simulink model "Mecanum_Mfunction_PID"  (R2022a)
settings: Solver=FixedStepAuto  StartTime=0.0  StopTime=20  FixedStep=0.001  RelTol=1e-3
values from neighbouring files (symbols this model uses):
  Cm = 0    [Mecanum_parameter_Mfunction_PID.m]
  Jm = 15.5*10^-7    (= 1.55e-06)    [Mecanum_parameter_Mfunction_PID.m]
  Kb = Kt    (= 0.0286)    [Mecanum_parameter_Mfunction_PID.m]
  Kf = 0    [Mecanum_parameter_Mfunction_PID.m]
  Kt = 28.6*10^-3    (= 0.0286)    [Mecanum_parameter_Mfunction_PID.m]
  La = 0.39*10^-3    (= 0.00039)    [Mecanum_parameter_Mfunction_PID.m]
  N = N_motor * N_wheel    (= 14)    [Mecanum_parameter_Mfunction_PID.m]
  Ra = 0.38    [Mecanum_parameter_Mfunction_PID.m]
libraries: simulink x1
(part 2 of 3)

== matlab function Mecanum_Mfunction_PID/Plant_Lagrange1/Lagrange_plant  ==
  settings: updateMethod=DISCRETE  sampleTime=0.001
  data: torque1 input; torque2 input; X_dotdot output; Y_dotdot output; Z_dotdot output; PHI_y_dotdot output; PHI_z_dotdot output; torque3 input; torque4 input; X_dot input; Y_dot input; Z_dot input; PHI_y_dot input; PHI_z_dot input; X input; Y input; Z input; PHI_y input; PHI_z input; X_dot output; Y_dot output; Z_dot output; PHI_y_dot output; PHI_z_dot output; X output; Y output; w1 input; w2 input; w3 input; w4 input; PHI_y output; PHI_z output
function [X_dotdot,Y_dotdot,Z_dotdot,PHI_y_dotdot,PHI_z_dotdot,X_dot,Y_dot,Z_dot,PHI_y_dot,PHI_z_dot,X,Y,PHI_y,PHI_z]  = fcn(torque1,torque2,torque3,torque4,X_dot,Y_dot,Z_dot,PHI_y_dot,PHI_z_dot,X,Y,Z,PHI_y,PHI_z,w1,w2,w3,w4)
%#codegen


%===== Parameter =====
%=== Body ===
m_b = 30; 
d = 0.6;
w = 0.4;
h = 1;
I_zb = 1/12*m_b*(d^2+w^2);
I_xb = 1/12*m_b*(h^2+d^2);
I_yb = 1/12*m_b*(w^2+h^2);

%=== Wheel ===
m_w = 0.4;
R = 0.05;
I_yw = m_w*R^2/2;
L_x_i = 0.2375;
L_y_i = 0.2394;
I_zw = m_w*(L_x_i^2+L_y_i^2);

%=== Friction ====
Friction = (m_b+4*m_w)/4*9.8*0.002;

if(w1>1)
    torque1 = torque1 - Friction;
else if(w1<-1)
    torque1 = torque1 + Friction;
    end
end

if(w2>1)
    torque2 = torque2 - Friction;
else if(w2<-1)
    torque2 = torque2 + Friction;
    end
end

if(w3>1)
    torque3 = torque3 - Friction;
else if(w3<-1)
    torque3 = torque3 + Friction;
    end
end

if(w4>1)
    torque4 = torque4 - Friction;
else if(w4<-1)
    torque4 = torque4 + Friction;
    end
end


dt = 0.001;
% 2D model

% Den_XY  = m_b + 4*m_w + 4*(I_yw/(R^2));
% Den_PHI = I_zb + 4*I_zw + 4*m_w*(Lx^2+Ly^2) + 4*I_yw/(R^2)*(Lx+Ly)^2 ;
% 
% Buff_X   = (cos(PHI)+sin(PHI))/R*(torque1+torque4) + (cos(PHI)-sin(PHI))/R*(torque2+torque3) - 4*I_yw/(R^2)*Y_dot*PHI_dot;
% Buff_Y   = (sin(PHI)-cos(PHI))/R*(torque1+torque4) + (sin(PHI)+cos(PHI))/R*(torque2+torque3) + 4*I_yw/(R^2)*X_dot*PHI_dot;
% Buff_PHI = (Lx+Ly)/R*(-torque1+torque2-torque3+torque4);

% X_dotdot   = Buff_X/Den_XY;
% Y_dotdot   = Buff_Y/Den_XY;
% PHI_dotdot = Buff_PHI/Den_PHI;
%%%%
X_dotdot = (32*G*I_yw^3*R^2*sin(2*PHI_y) - 32*G*I_yw^3*L_z_i^2*sin(2*PHI_y) + 8*G*I_yw^2*R^4*m_b*sin(2*PHI_y) + 32*G*I_yw^2*R^4*m_w*sin(2*PHI_y) + 16*I_yw^2*L_z_i^2*R^3*torque1*cos(PHI_z) + 16*I_yw^2*L_z_i^2*R^3*torque2*cos(PHI_z) + 16*I_yw^2*L_z_i^2*R^3*torque3*cos(PHI_z) + 16*I_yw^2*L_z_i^2*R^3*torque4*cos(PHI_z) + 64*I_yw^3*L_z_i^2*cos(PHI_y)*Y_dot*PHI_z_dot - 64*I_yw^3*R^2*cos(PHI_y)*Y_dot*PHI_z_dot + 32*G*I_yw^3*L_z_i^2*R^2*sin(2*PHI_y) - 64*I_yw^3*L_z_i^2*cos(PHI_y)^2*Z_dot*PHI_y_dot + 16*I_yw^2*R^3*torque1*cos(PHI_y)*cos(PHI_z) + 16*I_yw^2*R^3*torque2*cos(PHI_y)*cos(PHI_z) + 16*I_yw^2*R^3*torque3*cos(PHI_y)*cos(PHI_z) + 16*I_yw^2*R^3*torque4*cos(PHI_y)*cos(PHI_z) + 64*I_yw^3*R^2*cos(PHI_y)^2*Z_dot*PHI_y_dot - 32*I_yw^3*L_z_i^2*sin(2*PHI_y)*X_dot*PHI_y_dot + 32*I_yw^3*R^2*sin(2*PHI_y)*X_dot*PHI_y_dot + 16*I_yw^2*R^3*torque1*cos(PHI_y)*sin(PHI_z) - 16*I_yw^2*R^3*torque2*cos(PHI_y)*sin(PHI_z) - 16*I_yw^2*R^3*torque3*cos(PHI_y)*sin(PHI_z) + 16*I_yw^2*R^3*torque4*cos(PHI_y)*sin(PHI_z) + 8*G*I_yb*I_yw^2*R^2*sin(2*PHI_y) + 2*G*I_yb*I_yw*R^4*m_b*sin(2*PHI_y) + 8*G*I_yb*I_yw*R^4*m_w*sin(2*PHI_y) - 16*I_yw^2*L_z_i^2*R*torque1*cos(PHI_y)*sin(PHI_z) + 16*I_yw^2*L_z_i^2*R*torque2*cos(PHI_y)*sin(PHI_z) + 16*I_yw^2*L_z_i^2*R*torque3*cos(PHI_y)*sin(PHI_z) - 16*I_yw^2*L_z_i^2*R*torque4*cos(PHI_y)*sin(PHI_z) + 16*I_yw^2*L_z_i^2*R^3*torque1*cos(PHI_y)^2*cos(PHI_z)^3 + 16*I_yw^2*L_z_i^2*R^3*torque2*cos(PHI_y)^2*cos(PHI_z)^3 + 16*I_yw^2*L_z_i^2*R^3*torque3*cos(PHI_y)^2*cos(PHI_z)^3 + 16*I_yw^2*L_z_i^2*R^3*torque4*cos(PHI_y)^2*cos(PHI_z)^3 + 16*I_yw^2*R^4*m_b*cos(PHI_y)^2*Z_dot*PHI_y_dot + 64*I_yw^2*R^4*m_w*cos(PHI_y)^2*Z_dot*PHI_y_dot + 8*I_yw^2*R^4*m_b*sin(2*PHI_y)*X_dot*PHI_y_dot + 32*I_yw^2*R^4*m_w*sin(2*PHI_y)*X_dot*PHI_y_dot + 4*I_yw*L_z_i^2*R^5*m_b*torque1*cos(PHI_z) + 4*I_yw*L_z_i^2*R^5*m_b*torque2*cos(PHI_z) + 4*I_yw*L_z_i^2*R^5*m_b*torque3*cos(PHI_z) + 4*I_yw*L_z_i^2*R^5*m_b*torque4*cos(PHI_z) + 16*I_yw*L_z_i^2*R^5*m_w*torque1*cos(PHI_z) + 16*I_yw*L_z_i^2*R^5*m_w*torque2*cos(PHI_z) + 16*I_yw*L_z_i^2*R^5*m_w*torque3*cos(PHI_z) + 16*I_yw*L_z_i^2*R^5*m_w*torque4*cos(PHI_z) + 16*I_yw^2*L_z_i^2*R^3*torque1*cos(PHI_y)*cos(PHI_z) + 16*I_yw^2*L_z_i^2*R^3*torque2*cos(PHI_y)*cos(PHI_z) + 16*I_yw^2*L_z_i^2*R^3*torque3*cos(PHI_y)*cos(PHI_z) + 16*I_yw^2*L_z_i^2*R^3*torque4*cos(PHI_y)*cos(PHI_z) + 64*I_yw^3*L_z_i^2*R^2*cos(PHI_y)^2*Z_dot*PHI_y_dot - 64*I_yw^3*L_z_i^2*R^2*cos(PHI_z)^2*Y_dot*PHI_z_dot + 32*I_yw^3*L_z_i^2*R^2*sin(2*PHI_y)*X_dot*PHI_y_dot + 16*I_yw^2*L_z_i^2*R^3*torque1*cos(PHI_y)*sin(PHI_z) - 16*I_yw^2*L_z_i^2*R^3*torque2*cos(PHI_y)*sin(PHI_z) - 16*I_yw^2*L_z_i^2*R^3*torque3*cos(PHI_y)*sin(PHI_z) + 16*I_yw^2*L_z_i^2*R^3*torque4*cos(PHI_y)*sin(PHI_z) + 16*L_x_i^2*R^5*m_w^2*torque1*cos(PHI_y)*cos(PHI_z) + 16*L_x_i^2*R^5*m_w^2*torque2*cos(PHI_y)*cos(PHI_z) + 16*L_x_i^2*R^5*m_w^2*torque3*cos(PHI_y)*cos(PHI_z) + 16*L_x_i^2*R^5*m_w^2*torque4*cos(PHI_y)*cos(PHI_z) + 16*L_y_i^2*R^5*m_w^2*torque1*cos(PHI_y)*cos(PHI_z) + 16*L_y_i^2*R^5*m_w^2*torque2*cos(PHI_y)*cos(PHI_z) + 16*L_y_i^2*R^5*m_w^2*torque3*cos(PHI_y)*cos(PHI_z) + 16*L_y_i^2*R^5*m_w^2*torque4*cos(PHI_y)*cos(PHI_z) + 16*L_z_i^2*R^5*m_w^2*torque1*cos(PHI_y)*cos(PHI_z) + 16*L_z_i^2*R^5*m_w^2*torque2*cos(PHI_y)*cos(PHI_z) + 16*L_z_i^2*R^5*m_w^2*torque3*cos(PHI_y)*cos(PHI_z) + 16*L_z_i^2*R^5*m_w^2*torque4*cos(PHI_y)*cos(PHI_z) + 16*L_x_i^2*R^5*m_w^2*torque1*cos(PHI_y)*sin(PHI_z) - 16*L_x_i^2*R^5*m_w^2*torque2*cos(PHI_y)*sin(PHI_z) - 16*L_x_i^2*R^5*m_w^2*torque3*cos(PHI_y)*sin(PHI_z) + 16*L_x_i^2*R^5*m_w^2*torque4*cos(PHI_y)*sin(PHI_z) + 16*L_y_i^2*R^5*m_w^2*torque1*cos(PHI_y)*sin(PHI_z) - 16*L_y_i^2*R^5*m_w^2*torque2*cos(PHI_y)*sin(PHI_z) - 16*L_y_i^2*R^5*m_w^2*torque3*cos(PHI_y)*sin(PHI_z) + 16*L_y_i^2*R^5*m_w^2*torque4*cos(PHI_y)*sin(PHI_z) + 16*L_z_i^2*R^5*m_w^2*torque1*cos(PHI_y)*sin(PHI_z) - 16*L_z_i^2*R^5*m_w^2*torque2*cos(PHI_y)*sin(PHI_z) - 16*L_z_i^2*R^5*m_w^2*torque3*cos(PHI_y)*sin(PHI_z) + 16*L_z_i^2*R^5*m_w^2*torque4*cos(PHI_y)*sin(PHI_z) + 4*I_yb*I_yw*R^3*torque1*cos(PHI_y)*cos(PHI_z) + 4*I_yb*I_yw*R^3*torque2*cos(PHI_y)*cos(PHI_z) + 4*I_yb*I_yw*R^3*torque3*cos(PHI_y)*cos(PHI_z) + 4*I_yb*I_yw*R^3*torque4*cos(PHI_y)*cos(PHI_z) + 64*G*I_yw^3*L_z_i^2*R^2*cos(PHI_z)^2*sin(PHI_y) - 16*I_yb*I_yw^2*R^2*cos(PHI_y)*Y_dot*PHI_z_dot + 4*I_yb*I_yw*R^3*torque1*cos(PHI_y)*sin(PHI_z) - 4*I_yb*I_yw*R^3*torque2*cos(PHI_y)*sin(PHI_z) - 4*I_yb*I_yw*R^3*torque3*cos(PHI_y)*sin(PHI_z) + 4*I_yb*I_yw*R^3*torque4*cos(PHI_y)*sin(PHI_z) - 16*I_yw^2*L_z_i^2*R^3*torque1*cos(PHI_y)^2*cos(PHI_z) - 16*I_yw^2*L_z_i^2*R^3*torque1*cos(PHI_y)*cos(PHI_z)^3 - 16*I_yw^2*L_z_i^2*R^3*torque2*cos(PHI_y)^2*cos(PHI_z) - 16*I_yw^2*L_z_i^2*R^3*torque2*cos(PHI_y)*cos(PHI_z)^3 - 16*I_yw^2*L_z_i^2*R^3*torque3*cos(PHI_y)^2*cos(PHI_z) - 16*I_yw^2*L_z_i^2*R^3*torque3*cos(PHI_y)*cos(PHI_z)^3 - 16*I_yw^2*L_z_i^2*R^3*torque4*cos(PHI_y)^2*cos(PHI_z) - 16*I_yw^2*L_z_i^2*R^3*torque4*cos(PHI_y)*cos(PHI_z)^3 + I_yb*R^5*m_b*torque1*cos(PHI_y)*cos(PHI_z) + I_yb*R^5*m_b*torque2*cos(PHI_y)*cos(PHI_z) + I_yb*R^5*m_b*torque3*cos(PHI_y)*cos(PHI_z) + I_yb*R^5*m_b*torque4*cos(PHI_y)*cos(PHI_z) + 4*I_yw*R^5*m_b*torque1*cos(PHI_y)*cos(PHI_z) + 4*I_yw*R^5*m_b*torque2*cos(PHI_y)*cos(PHI_z) + 4*I_yw*R^5*m_b*torque3*cos(PHI_y)*cos(PHI_z) + 4*I_yw*R^5*m_b*torque4*cos(PHI_y)*cos(PHI_z) + 4*I_yb*R^5*m_w*torque1*cos(PHI_y)*cos(PHI_z) + 4*I_yb*R^5*m_w*torque2*cos(PHI_y)*cos(PHI_z) + 4*I_yb*R^5*m_w*torque3*cos(PHI_y)*cos(PHI_z) + 4*I_yb*R^5*m_w*torque4*cos(PHI_y)*cos(PHI_z) + 16*I_yw*R^5*m_w*torque1*cos(PHI_y)*cos(PHI_z) + 16*I_yw*R^5*m_w*torque2*cos(PHI_y)*cos(PHI_z) + 16*I_yw*R^5*m_w*torque3*cos(PHI_y)*cos(PHI_z) + 16*I_yw*R^5*m_w*torque4*cos(PHI_y)*cos(PHI_z) - 16*I_yw^2*R^4*m_b*cos(PHI_y)*Y_dot*PHI_z_dot - 64*I_yw^2*R^4*m_w*cos(PHI_y)*Y_dot*PHI_z_dot - 8*G*I_yw^2*L_z_i^2*R^2*m_b*sin(2*PHI_y) + 32*G*I_yw^2*L_x_i^2*R^2*m_w*sin(2*PHI_y) + 32*G*I_yw*L_x_i^2*R^4*m_w^2*sin(2*PHI_y) + 32*G*I_yw^2*L_y_i^2*R^2*m_w*sin(2*PHI_y) + 32*G*I_yw*L_y_i^2*R^4*m_w^2*sin(2*PHI_y) + 32*G*I_yw*L_z_i^2*R^4*m_w^2*sin(2*PHI_y) + I_yb*R^5*m_b*torque1*cos(PHI_y)*sin(PHI_z) - I_yb*R^5*m_b*torque2*cos(PHI_y)*sin(PHI_z) - I_yb*R^5*m_b*torque3*cos(PHI_y)*sin(PHI_z) + I_yb*R^5*m_b*torque4*cos(PHI_y)*sin(PHI_z) + 4*I_yw*R^5*m_b*torque1*cos(PHI_y)*sin(PHI_z) - 4*I_yw*R^5*m_b*torque2*cos(PHI_y)*sin(PHI_z) - 4*I_yw*R^5*m_b*torque3*cos(PHI_y)*sin(PHI_z) + 4*I_yw*R^5*m_b*torque4*cos(PHI_y)*sin(PHI_z) + 4*I_yb*R^5*m_w*torque1*cos(PHI_y)*sin(PHI_z) - 4*I_yb*R^5*m_w*torque2*cos(PHI_y)*sin(PHI_z) - 4*I_yb*R^5*m_w*torque3*cos(PHI_y)*sin(PHI_z) + 4*I_yb*R^5*m_w*torque4*cos(PHI_y)*sin(PHI_z) + 16*I_yw*R^5*m_w*torque1*cos(PHI_y)*sin(PHI_z) - 16*I_yw*R^5*m_w*torque2*cos(PHI_y)*sin(PHI_z) - 16*I_yw*R^5*m_w*torque3*cos(PHI_y)*sin(PHI_z) + 16*I_yw*R^5*m_w*torque4*cos(PHI_y)*sin(PHI_z) + 16*I_yb*I_yw^2*R^2*cos(PHI_y)^2*Z_dot*PHI_y_dot - 16*I_yw^2*L_z_i^2*R*torque1*cos(PHI_y)*cos(PHI_z) - 16*I_yw^2*L_z_i^2*R*torque2*cos(PHI_y)*cos(PHI_z) - 16*I_yw^2*L_z_i^2*R*torque3*cos(PHI_y)*cos(PHI_z) - 16*I_yw^2*L_z_i^2*R*torque4*cos(PHI_y)*cos(PHI_z) - 64*I_yw^3*L_z_i^2*R^2*cos(PHI_y)*Y_dot*PHI_z_dot + 8*I_yb*I_yw^2*R^2*sin(2*PHI_y)*X_dot*PHI_y_dot - 16*I_yw^2*L_z_i^2*R^3*torque1*cos(PHI_y)*cos(PHI_z)^2*sin(PHI_z) + 16*I_yw^2*L_z_i^2*R^3*torque2*cos(PHI_y)*cos(PHI_z)^2*sin(PHI_z) + 16*I_yw^2*L_z_i^2*R^3*torque3*cos(PHI_y)*cos(PHI_z)^2*sin(PHI_z) - 16*I_yw^2*L_z_i^2*R^3*torque4*cos(PHI_y)*cos(PHI_z)^2*sin(PHI_z) + 16*G*I_yw^2*L_z_i^2*R^4*m_b*cos(PHI_z)^2*sin(PHI_y) + 64*G*I_yw^2*L_z_i^2*R^4*m_w*cos(PHI_z)^2*sin(PHI_y) + 2*I_yb*I_yw*R^4*m_b*sin(2*PHI_y)*X_dot*PHI_y_dot + 8*I_yb*I_yw*R^4*m_w*sin(2*PHI_y)*X_dot*PHI_y_dot + 16*I_yw^2*L_z_i^2*R^3*torque1*cos(PHI_y)^2*cos(PHI_z)^2*sin(PHI_z) - 16*I_yw^2*L_z_i^2*R^3*torque2*cos(PHI_y)^2*cos(PHI_z)^2*sin(PHI_z) - 16*I_yw^2*L_z_i^2*R^3*torque3*cos(PHI_y)^2*cos(PHI_z)^2*sin(PHI_z) + 16*I_yw^2*L_z_i^2*R^3*torque4*cos(PHI_y)^2*cos(PHI_z)^2*sin(PHI_z) - 4*I_yw*L_z_i^2*R^3*m_b*torque1*cos(PHI_y)*cos(PHI_z) - 4*I_yw*L_z_i^2*R^3*m_b*torque2*cos(PHI_y)*cos(PHI_z) - 4*I_yw*L_z_i^2*R^3*m_b*torque3*cos(PHI_y)*cos(PHI_z) - 4*I_yw*L_z_i^2*R^3*m_b*torque4*cos(PHI_y)*cos(PHI_z) + 16*I_yw*L_x_i^2*R^3*m_w*torque1*cos(PHI_y)*cos(PHI_z) + 16*I_yw*L_x_i^2*R^3*m_w*torque2*cos(PHI_y)*cos(PHI_z) + 16*I_yw*L_x_i^2*R^3*m_w*torque3*cos(PHI_y)*cos(PHI_z) + 16*I_yw*L_x_i^2*R^3*m_w*torque4*cos(PHI_y)*cos(PHI_z) + 16*I_yw*L_y_i^2*R^3*m_w*torque1*cos(PHI_y)*cos(PHI_z) + 16*I_yw*L_y_i^2*R^3*m_w*torque2*cos(PHI_y)*cos(PHI_z) + 16*I_yw*L_y_i^2*R^3*m_w*torque3*cos(PHI_y)*cos(PHI_z) + 16*I_yw*L_y_i^2*R^3*m_w*torque4*cos(PHI_y)*cos(PHI_z) + 16*I_yw^2*L_z_i^2*R^2*m_b*cos(PHI_y)*Y_dot*PHI_z_dot - 64*I_yw^2*L_x_i^2*R^2*m_w*cos(PHI_y)*Y_dot*PHI_z_dot - 64*I_yw*L_x_i^2*R^4*m_w^2*cos(PHI_y)*Y_dot*PHI_z_dot - 64*I_yw^2*L_y_i^2*R^2*m_w*cos(PHI_y)*Y_dot*PHI_z_dot - 64*I_yw*L_y_i^2*R^4*m_w^2*cos(PHI_y)*Y_dot*PHI_z_dot - 64*I_yw*L_z_i^2*R^4*m_w^2*cos(PHI_y)*Y_dot*PHI_z_dot - 4*I_yw*L_z_i^2*R^3*m_b*torque1*cos(PHI_y)*sin(PHI_z) + 4*I_yw*L_z_i^2*R^3*m_b*torque2*cos(PHI_y)*sin(PHI_z) + 4*I_yw*L_z_i^2*R^3*m_b*torque3*cos(PHI_y)*sin(PHI_z) - 4*I_yw*L_z_i^2*R^3*m_b*torque4*cos(PHI_y)*sin(PHI_z) + 16*I_yw*L_x_i^2*R^3*m_w*torque1*cos(PHI_y)*sin(PHI_z) - 16*I_yw*L_x_i^2*R^3*m_w*torque2*cos(PHI_y)*sin(PHI_z) - 16*I_yw*L_x_i^2*R^3*m_w*torque3*cos(PHI_y)*sin(PHI_z) + 16*I_yw*L_x_i^2*R^3*m_w*torque4*cos(PHI_y)*sin(PHI_z) + 16*I_yw*L_y_i^2*R^3*m_w*torque1*cos(PHI_y)*sin(PHI_z) - 16*I_yw*L_y_i^2*R^3*m_w*torque2*cos(PHI_y)*sin(PHI_z) - 16*I_yw*L_y_i^2*R^3*m_w*torque3*cos(PHI_y)*sin(PHI_z) + 16*I_yw*L_y_i^2*R^3*m_w*torque4*cos(PHI_y)*sin(PHI_z) + 4*L_x_i^2*R^5*m_b*m_w*torque1*cos(PHI_y)*cos(PHI_z) + 4*L_x_i^2*R^5*m_b*m_w*torque2*cos(PHI_y)*cos(PHI_z) + 4*L_x_i^2*R^5*m_b*m_w*torque3*cos(PHI_y)*cos(PHI_z) + 4*L_x_i^2*R^5*m_b*m_w*torque4*cos(PHI_y)*cos(PHI_z) + 4*L_y_i^2*R^5*m_b*m_w*torque1*cos(PHI_y)*cos(PHI_z) + 4*L_y_i^2*R^5*m_b*m_w*torque2*cos(PHI_y)*cos(PHI_z) + 4*L_y_i^2*R^5*m_b*m_w*torque3*cos(PHI_y)*cos(PHI_z) + 4*L_y_i^2*R^5*m_b*m_w*torque4*cos(PHI_y)*cos(PHI_z) + 4*L_z_i^2*R^5*m_b*m_w*torque1*cos(PHI_y)*cos(PHI_z) + 4*L_z_i^2*R^5*m_b*m_w*torque2*cos(PHI_y)*cos(PHI_z) + 4*L_z_i^2*R^5*m_b*m_w*torque3*cos(PHI_y)*cos(PHI_z) + 4*L_z_i^2*R^5*m_b*m_w*torque4*cos(PHI_y)*cos(PHI_z) + 64*I_yw^3*L_z_i^2*R^2*cos(PHI_y)*cos(PHI_z)^2*Z_dot*PHI_y_dot + 4*L_x_i^2*R^5*m_b*m_w*torque1*cos(PHI_y)*sin(PHI_z) - 4*L_x_i^2*R^5*m_b*m_w*torque2*cos(PHI_y)*sin(PHI_z) - 4*L_x_i^2*R^5*m_b*m_w*torque3*cos(PHI_y)*sin(PHI_z) + 4*L_x_i^2*R^5*m_b*m_w*torque4*cos(PHI_y)*sin(PHI_z) + 4*L_y_i^2*R^5*m_b*m_w*torque1*cos(PHI_y)*sin(PHI_z) - 4*L_y_i^2*R^5*m_b*m_w*torque2*cos(PHI_y)*sin(PHI_z) - 4*L_y_i^2*R^5*m_b*m_w*torque3*cos(PHI_y)*sin(PHI_z) + 4*L_y_i^2*R^5*m_b*m_w*torque4*cos(PHI_y)*sin(PHI_z) + 4*L_z_i^2*R^5*m_b*m_w*torque1*cos(PHI_y)*sin(PHI_z) - 4*L_z_i^2*R^5*m_b*m_w*torque2*cos(PHI_y)*sin(PHI_z) - 4*L_z_i^2*R^5*m_b*m_w*torque3*cos(PHI_y)*sin(PHI_z) + 4*L_z_i^2*R^5*m_b*m_w*torque4*cos(PHI_y)*sin(PHI_z) + 64*I_yw^3*L_z_i^2*R^2*cos(PHI_y)*cos(PHI_z)^2*Y_dot*PHI_z_dot + 16*I_yw^2*L_z_i^2*R^3*torque1*cos(PHI_y)*cos(PHI_z)*sin(PHI_y) + 16*I_yw^2*L_z_i^2*R^3*torque2*cos(PHI_y)*cos(PHI_z)*sin(PHI_y) + 16*I_yw^2*L_z_i^2*R^3*torque3*cos(PHI_y)*cos(PHI_z)*sin(PHI_y) + 16*I_yw^2*L_z_i^2*R^3*torque4*cos(PHI_y)*cos(PHI_z)*sin(PHI_y) + 64*I_yw^3*L_z_i^2*R^2*cos(PHI_z)^2*sin(PHI_y)*X_dot*PHI_y_dot - 4*I_yb*I_yw*R^4*m_b*cos(PHI_y)*Y_dot*PHI_z_dot - 16*I_yb*I_yw*R^4*m_w*cos(PHI_y)*Y_dot*PHI_z_dot - 16*I_yw^2*L_z_i^2*R^2*m_b*cos(PHI_y)^2*Z_dot*PHI_y_dot + 64*I_yw^2*L_x_i^2*R^2*m_w*cos(PHI_y)^2*Z_dot*PHI_y_dot + 64*I_yw*L_x_i^2*R^4*m_w^2*cos(PHI_y)^2*Z_dot*PHI_y_dot + 64*I_yw^2*L_y_i^2*R^2*m_w*cos(PHI_y)^2*Z_dot*PHI_y_dot + 64*I_yw*L_y_i^2*R^4*m_w^2*cos(PHI_y)^2*Z_dot*PHI_y_dot + 64*I_yw*L_z_i^2*R^4*m_w^2*cos(PHI_y)^2*Z_dot*PHI_y_dot - 16*I_yw^2*L_z_i^2*R^4*m_b*cos(PHI_z)^2*Y_dot*PHI_z_dot - 64*I_yw^2*L_z_i^2*R^4*m_w*cos(PHI_z)^2*Y_dot*PHI_z_dot - 64*G*I_yw^3*L_z_i^2*R^2*cos(PHI_y)*cos(PHI_z)^2*sin(PHI_y) - 8*I_yw^2*L_z_i^2*R^2*m_b*sin(2*PHI_y)*X_dot*PHI_y_dot + 32*I_yw^2*L_x_i^2*R^2*m_w*sin(2*PHI_y)*X_dot*PHI_y_dot + 32*I_yw*L_x_i^2*R^4*m_w^2*sin(2*PHI_y)*X_dot*PHI_y_dot + 32*I_yw^2*L_y_i^2*R^2*m_w*sin(2*PHI_y)*X_dot*PHI_y_dot + 32*I_yw*L_y_i^2*R^4*m_w^2*sin(2*PHI_y)*X_dot*PHI_y_dot + 32*I_yw*L_z_i^2*R^4*m_w^2*sin(2*PHI_y)*X_dot*PHI_y_dot + 8*G*I_yw*L_x_i^2*R^4*m_b*m_w*sin(2*PHI_y) + 8*G*I_yw*L_y_i^2*R^4*m_b*m_w*sin(2*PHI_y) + 8*G*I_yw*L_z_i^2*R^4*m_b*m_w*sin(2*PHI_y) - 64*I_yw^3*L_z_i^2*R^2*cos(PHI_y)^2*cos(PHI_z)^2*Z_dot*PHI_y_dot - 16*I_yw^2*L_z_i^2*R^3*torque1*cos(PHI_y)*cos(PHI_z)^3*sin(PHI_y) - 16*I_yw^2*L_z_i^2*R^3*torque2*cos(PHI_y)*cos(PHI_z)^3*sin(PHI_y) - 16*I_yw^2*L_z_i^2*R^3*torque3*cos(PHI_y)*cos(PHI_z)^3*sin(PHI_y) - 16*I_yw^2*L_z_i^2*R^3*torque4*cos(PHI_y)*cos(PHI_z)^3*sin(PHI_y) + 4*I_yb*I_yw*R^4*m_b*cos(PHI_y)^2*Z_dot*PHI_y_dot + 16*I_yb*I_yw*R^4*m_w*cos(PHI_y)^2*Z_dot*PHI_y_dot + 16*I_yw^2*L_z_i^2*R^4*m_b*cos(PHI_y)*cos(PHI_z)^2*Z_dot*PHI_y_dot + 64*I_yw^2*L_z_i^2*R^4*m_w*cos(PHI_y)*cos(PHI_z)^2*Z_dot*PHI_y_dot + 16*I_yw^2*L_z_i^2*R^4*m_b*cos(PHI_z)^2*sin(PHI_y)*X_dot*PHI_y_dot + 64*I_yw^2*L_z_i^2*R^4*m_w*cos(PHI_z)^2*sin(PHI_y)*X_dot*PHI_y_dot - 16*I_yw^2*L_z_i^2*R^3*torque1*cos(PHI_y)*cos(PHI_z)^2*sin(PHI_y)*sin(PHI_z) + 16*I_yw^2*L_z_i^2*R^3*torque2*cos(PHI_y)*cos(PHI_z)^2*sin(PHI_y)*sin(PHI_z) + 16*I_yw^2*L_z_i^2*R^3*torque3*cos(PHI_y)*cos(PHI_z)^2*sin(PHI_y)*sin(PHI_z) - 16*I_yw^2*L_z_i^2*R^3*torque4*cos(PHI_y)*cos(PHI_z)^2*sin(PHI_y)*sin(PHI_z) - 16*I_yw*L_x_i^2*R^4*m_b*m_w*cos(PHI_y)*Y_dot*PHI_z_dot - 16*I_yw*L_y_i^2*R^4*m_b*m_w*cos(PHI_y)*Y_dot*PHI_z_dot - 16*I_yw*L_z_i^2*R^4*m_b*m_w*cos(PHI_y)*Y_dot*PHI_z_dot + 64*I_yw^3*L_z_i^2*R^2*cos(PHI_y)*cos(PHI_z)*sin(PHI_z)*X_dot*PHI_z_dot - 64*I_yw^3*L_z_i^2*R^2*cos(PHI_y)*cos(PHI_z)*sin(PHI_z)*Z_dot*PHI_z_dot - 64*I_yw^3*L_z_i^2*R^2*cos(PHI_z)*sin(PHI_y)*sin(PHI_z)*Z_dot*PHI_z_dot + 16*I_yw*L_x_i^2*R^4*m_b*m_w*cos(PHI_y)^2*Z_dot*PHI_y_dot + 16*I_yw*L_y_i^2*R^4*m_b*m_w*cos(PHI_y)^2*Z_dot*PHI_y_dot + 16*I_yw*L_z_i^2*R^4*m_b*m_w*cos(PHI_y)^2*Z_dot*PHI_y_dot - 64*I_yw^3*L_z_i^2*R^2*cos(PHI_y)*cos(PHI_z)^2*sin(PHI_y)*X_dot*PHI_y_dot + 8*I_yw*L_x_i^2*R^4*m_b*m_w*sin(2*PHI_y)*X_dot*PHI_y_dot + 8*I_yw*L_y_i^2*R^4*m_b*m_w*sin(2*PHI_y)*X_dot*PHI_y_dot + 8*I_yw*L_z_i^2*R^4*m_b*m_w*sin(2*PHI_y)*X_dot*PHI_y_dot - 64*I_yw^3*L_z_i^2*R^2*cos(PHI_y)^3*cos(PHI_z)*sin(PHI_z)*X_dot*PHI_z_dot + 64*I_yw^3*L_z_i^2*R^2*cos(PHI_y)^3*cos(PHI_z)*sin(PHI_z)*Z_dot*PHI_z_dot - 16*I_yw^2*L_z_i^2*R^4*m_b*cos(PHI_z)*sin(PHI_y)*sin(PHI_z)*Z_dot*PHI_z_dot - 64*I_yw^2*L_z_i^2*R^4*m_w*cos(PHI_z)*sin(PHI_y)*sin(PHI_z)*Z_dot*PHI_z_dot + 64*I_yw^3*L_z_i^2*R^2*cos(PHI_y)^2*cos(PHI_z)*sin(PHI_y)*sin(PHI_z)*X_dot*PHI_z_dot + 64*I_yw^3*L_z_i^2*R^2*cos(PHI_y)^2*cos(PHI_z)*sin(PHI_y)*sin(PHI_z)*Z_dot*PHI_z_dot + 16*I_yw^2*L_z_i^2*R^4*m_b*cos(PHI_y)*cos(PHI_z)*sin(PHI_z)*X_dot*PHI_z_dot + 64*I_yw^2*L_z_i^2*R^4*m_w*cos(PHI_y)*cos(PHI_z)*sin(PHI_z)*X_dot*PHI_z_dot)/((4*I_yw + R^2*m_b + 4*R^2*m_w)*(16*I_yw^2*R^2 - 16*I_yw^2*L_z_i^2 + 16*I_yw^2*L_z_i^2*R^2 + 16*L_x_i^2*R^4*m_w^2 + 16*L_y_i^2*R^4*m_w^2 + 16*L_z_i^2*R^4*m_w^2 + 4*I_yb*I_yw*R^2 + I_yb*R^4*m_b + 4*I_yw*R^4*m_b + 4*I_yb*R^4*m_w + 16*I_yw*R^4*m_w - 16*I_yw^2*L_z_i^2*R^2*cos(PHI_z)^2 - 4*I_yw*L_z_i^2*R^2*m_b + 16*I_yw*L_x_i^2*R^2*m_w + 16*I_yw*L_y_i^2*R^2*m_w + 4*L_x_i^2*R^4*m_b*m_w + 4*L_y_i^2*R^4*m_b*m_w + 4*L_z_i^2*R^4*m_b*m_w + 16*I_yw^2*L_z_i^2*R^2*cos(PHI_y)*cos(PHI_z)^2 - 16*I_yw^2*L_z_i^2*R^2*cos(PHI_z)^2*sin(PHI_y)));
Y_dotdot = (16*I_yw^2*R^3*torque2*cos(PHI_z) - 16*I_yw^2*R^3*torque1*cos(PHI_z) + 16*I_yw^2*R^3*torque3*cos(PHI_z) - 16*I_yw^2*R^3*torque4*cos(PHI_z) + 16*I_yw^2*R^3*torque1*sin(PHI_z) + 16*I_yw^2*R^3*torque2*sin(PHI_z) + 16*I_yw^2*R^3*torque3*sin(PHI_z) + 16*I_yw^2*R^3*torque4*sin(PHI_z) - 16*I_yw^2*L_z_i^2*R^3*torque1*cos(PHI_z) + 16*I_yw^2*L_z_i^2*R^3*torque2*cos(PHI_z) + 16*I_yw^2*L_z_i^2*R^3*torque3*cos(PHI_z) - 16*I_yw^2*L_z_i^2*R^3*torque4*cos(PHI_z) - 16*L_x_i^2*R^5*m_w^2*torque1*cos(PHI_z) + 16*L_x_i^2*R^5*m_w^2*torque2*cos(PHI_z) + 16*L_x_i^2*R^5*m_w^2*torque3*cos(PHI_z) - 16*L_x_i^2*R^5*m_w^2*torque4*cos(PHI_z) - 16*L_y_i^2*R^5*m_w^2*torque1*cos(PHI_z) + 16*L_y_i^2*R^5*m_w^2*torque2*cos(PHI_z) + 16*L_y_i^2*R^5*m_w^2*torque3*cos(PHI_z) - 16*L_y_i^2*R^5*m_w^2*torque4*cos(PHI_z) - 16*L_z_i^2*R^5*m_w^2*torque1*cos(PHI_z) + 16*L_z_i^2*R^5*m_w^2*torque2*cos(PHI_z) + 16*L_z_i^2*R^5*m_w^2*torque3*cos(PHI_z) - 16*L_z_i^2*R^5*m_w^2*torque4*cos(PHI_z) - 64*I_yw^3*L_z_i^2*cos(PHI_y)*X_dot*PHI_z_dot + 64*I_yw^3*R^2*cos(PHI_y)*X_dot*PHI_z_dot + 16*L_x_i^2*R^5*m_w^2*torque1*sin(PHI_z) + 16*L_x_i^2*R^5*m_w^2*torque2*sin(PHI_z) + 16*L_x_i^2*R^5*m_w^2*torque3*sin(PHI_z) + 16*L_x_i^2*R^5*m_w^2*torque4*sin(PHI_z) + 16*L_y_i^2*R^5*m_w^2*torque1*sin(PHI_z) + 16*L_y_i^2*R^5*m_w^2*torque2*sin(PHI_z) + 16*L_y_i^2*R^5*m_w^2*torque3*sin(PHI_z) + 16*L_y_i^2*R^5*m_w^2*torque4*sin(PHI_z) + 16*L_z_i^2*R^5*m_w^2*torque1*sin(PHI_z) + 16*L_z_i^2*R^5*m_w^2*torque2*sin(PHI_z) + 16*L_z_i^2*R^5*m_w^2*torque3*sin(PHI_z) + 16*L_z_i^2*R^5*m_w^2*torque4*sin(PHI_z) - 4*I_yb*I_yw*R^3*torque1*cos(PHI_z) + 4*I_yb*I_yw*R^3*torque2*cos(PHI_z) + 4*I_yb*I_yw*R^3*torque3*cos(PHI_z) - 4*I_yb*I_yw*R^3*torque4*cos(PHI_z) + 64*I_yw^3*L_z_i^2*sin(PHI_y)*Z_dot*PHI_z_dot - 64*I_yw^3*R^2*sin(PHI_y)*Z_dot*PHI_z_dot + 4*I_yb*I_yw*R^3*torque1*sin(PHI_z) + 4*I_yb*I_yw*R^3*torque2*sin(PHI_z) + 4*I_yb*I_yw*R^3*torque3*sin(PHI_z) + 4*I_yb*I_yw*R^3*torque4*sin(PHI_z) + 16*I_yw^2*L_z_i^2*R^3*torque1*cos(PHI_z)^3 - 16*I_yw^2*L_z_i^2*R^3*torque2*cos(PHI_z)^3 - 16*I_yw^2*L_z_i^2*R^3*torque3*cos(PHI_z)^3 + 16*I_yw^2*L_z_i^2*R^3*torque4*cos(PHI_z)^3 - I_yb*R^5*m_b*torque1*cos(PHI_z) + I_yb*R^5*m_b*torque2*cos(PHI_z) + I_yb*R^5*m_b*torque3*cos(PHI_z) - I_yb*R^5*m_b*torque4*cos(PHI_z) - 4*I_yw*R^5*m_b*torque1*cos(PHI_z) + 4*I_yw*R^5*m_b*torque2*cos(PHI_z) + 4*I_yw*R^5*m_b*torque3*cos(PHI_z) - 4*I_yw*R^5*m_b*torque4*cos(PHI_z) - 4*I_yb*R^5*m_w*torque1*cos(PHI_z) + 4*I_yb*R^5*m_w*torque2*cos(PHI_z) + 4*I_yb*R^5*m_w*torque3*cos(PHI_z) - 4*I_yb*R^5*m_w*torque4*cos(PHI_z) - 16*I_yw*R^5*m_w*torque1*cos(PHI_z) + 16*I_yw*R^5*m_w*torque2*cos(PHI_z) + 16*I_yw*R^5*m_w*torque3*cos(PHI_z) - 16*I_yw*R^5*m_w*torque4*cos(PHI_z) + 16*I_yw^2*L_z_i^2*R^3*torque1*sin(PHI_z)^3 + 16*I_yw^2*L_z_i^2*R^3*torque2*sin(PHI_z)^3 + 16*I_yw^2*L_z_i^2*R^3*torque3*sin(PHI_z)^3 + 16*I_yw^2*L_z_i^2*R^3*torque4*sin(PHI_z)^3 + I_yb*R^5*m_b*torque1*sin(PHI_z) + I_yb*R^5*m_b*torque2*sin(PHI_z) + I_yb*R^5*m_b*torque3*sin(PHI_z) + I_yb*R^5*m_b*torque4*sin(PHI_z) + 4*I_yw*R^5*m_b*torque1*sin(PHI_z) + 4*I_yw*R^5*m_b*torque2*sin(PHI_z) + 4*I_yw*R^5*m_b*torque3*sin(PHI_z) + 4*I_yw*R^5*m_b*torque4*sin(PHI_z) + 4*I_yb*R^5*m_w*torque1*sin(PHI_z) + 4*I_yb*R^5*m_w*torque2*sin(PHI_z) + 4*I_yb*R^5*m_w*torque3*sin(PHI_z) + 4*I_yb*R^5*m_w*torque4*sin(PHI_z) + 16*I_yw*R^5*m_w*torque1*sin(PHI_z) + 16*I_yw*R^5*m_w*torque2*sin(PHI_z) + 16*I_yw*R^5*m_w*torque3*sin(PHI_z) + 16*I_yw*R^5*m_w*torque4*sin(PHI_z) + 16*I_yw^2*L_z_i^2*R*torque1*cos(PHI_z) - 16*I_yw^2*L_z_i^2*R*torque2*cos(PHI_z) - 16*I_yw^2*L_z_i^2*R*torque3*cos(PHI_z) + 16*I_yw^2*L_z_i^2*R*torque4*cos(PHI_z) - 16*I_yw^2*L_z_i^2*R*torque1*sin(PHI_z) - 16*I_yw^2*L_z_i^2*R*torque2*sin(PHI_z) - 16*I_yw^2*L_z_i^2*R*torque3*sin(PHI_z) - 16*I_yw^2*L_z_i^2*R*torque4*sin(PHI_z) - 64*I_yw^3*L_z_i^2*R^2*sin(PHI_y)*Z_dot*PHI_z_dot + 4*I_yw*L_z_i^2*R^3*m_b*torque1*cos(PHI_z) - 4*I_yw*L_z_i^2*R^3*m_b*torque2*cos(PHI_z) - 4*I_yw*L_z_i^2*R^3*m_b*torque3*cos(PHI_z) + 4*I_yw*L_z_i^2*R^3*m_b*torque4*cos(PHI_z) - 16*I_yw*L_x_i^2*R^3*m_w*torque1*cos(PHI_z) + 16*I_yw*L_x_i^2*R^3*m_w*torque2*cos(PHI_z) + 16*I_yw*L_x_i^2*R^3*m_w*torque3*cos(PHI_z) - 16*I_yw*L_x_i^2*R^3*m_w*torque4*cos(PHI_z) - 16*I_yw*L_y_i^2*R^3*m_w*torque1*cos(PHI_z) + 16*I_yw*L_y_i^2*R^3*m_w*torque2*cos(PHI_z) + 16*I_yw*L_y_i^2*R^3*m_w*torque3*cos(PHI_z) - 16*I_yw*L_y_i^2*R^3*m_w*torque4*cos(PHI_z) - 4*I_yw*L_z_i^2*R^3*m_b*torque1*sin(PHI_z) - 4*I_yw*L_z_i^2*R^3*m_b*torque2*sin(PHI_z) - 4*I_yw*L_z_i^2*R^3*m_b*torque3*sin(PHI_z) + 4*I_yw*L_z_i^2*R^5*m_b*torque1*sin(PHI_z) - 4*I_yw*L_z_i^2*R^3*m_b*torque4*sin(PHI_z) + 4*I_yw*L_z_i^2*R^5*m_b*torque2*sin(PHI_z) + 4*I_yw*L_z_i^2*R^5*m_b*torque3*sin(PHI_z) + 4*I_yw*L_z_i^2*R^5*m_b*torque4*sin(PHI_z) + 16*I_yw*L_x_i^2*R^3*m_w*torque1*sin(PHI_z) + 16*I_yw*L_x_i^2*R^3*m_w*torque2*sin(PHI_z) + 16*I_yw*L_x_i^2*R^3*m_w*torque3*sin(PHI_z) + 16*I_yw*L_x_i^2*R^3*m_w*torque4*sin(PHI_z) + 16*I_yw*L_y_i^2*R^3*m_w*torque1*sin(PHI_z) + 16*I_yw*L_y_i^2*R^3*m_w*torque2*sin(PHI_z) + 16*I_yw*L_y_i^2*R^3*m_w*torque3*sin(PHI_z) + 16*I_yw*L_y_i^2*R^3*m_w*torque4*sin(PHI_z) + 16*I_yw*L_z_i^2*R^5*m_w*torque1*sin(PHI_z) + 16*I_yw*L_z_i^2*R^5*m_w*torque2*sin(PHI_z) + 16*I_yw*L_z_i^2*R^5*m_w*torque3*sin(PHI_z) + 16*I_yw*L_z_i^2*R^5*m_w*torque4*sin(PHI_z) - 4*L_x_i^2*R^5*m_b*m_w*torque1*cos(PHI_z) + 4*L_x_i^2*R^5*m_b*m_w*torque2*cos(PHI_z) + 4*L_x_i^2*R^5*m_b*m_w*torque3*cos(PHI_z) - 4*L_x_i^2*R^5*m_b*m_w*torque4*cos(PHI_z) - 4*L_y_i^2*R^5*m_b*m_w*torque1*cos(PHI_z) + 4*L_y_i^2*R^5*m_b*m_w*torque2*cos(PHI_z) + 4*L_y_i^2*R^5*m_b*m_w*torque3*cos(PHI_z) - 4*L_y_i^2*R^5*m_b*m_w*torque4*cos(PHI_z) - 4*L_z_i^2*R^5*m_b*m_w*torque1*cos(PHI_z) + 4*L_z_i^2*R^5*m_b*m_w*torque2*cos(PHI_z) + 4*L_z_i^2*R^5*m_b*m_w*torque3*cos(PHI_z) - 4*L_z_i^2*R^5*m_b*m_w*torque4*cos(PHI_z) + 4*L_x_i^2*R^5*m_b*m_w*torque1*sin(PHI_z) + 4*L_x_i^2*R^5*m_b*m_w*torque2*sin(PHI_z) + 4*L_x_i^2*R^5*m_b*m_w*torque3*sin(PHI_z) + 4*L_x_i^2*R^5*m_b*m_w*torque4*sin(PHI_z) + 4*L_y_i^2*R^5*m_b*m_w*torque1*sin(PHI_z) + 4*L_y_i^2*R^5*m_b*m_w*torque2*sin(PHI_z) + 4*L_y_i^2*R^5*m_b*m_w*torque3*sin(PHI_z) + 4*L_y_i^2*R^5*m_b*m_w*torque4*sin(PHI_z) + 4*L_z_i^2*R^5*m_b*m_w*torque1*sin(PHI_z) + 4*L_z_i^2*R^5*m_b*m_w*torque2*sin(PHI_z) + 4*L_z_i^2*R^5*m_b*m_w*torque3*sin(PHI_z) + 4*L_z_i^2*R^5*m_b*m_w*torque4*sin(PHI_z) + 64*I_yw^3*L_z_i^2*R^2*cos(PHI_z)^2*Z_dot*PHI_z_dot - 16*I_yw^2*L_z_i^2*R^3*torque1*sin(PHI_y)*sin(PHI_z) - 16*I_yw^2*L_z_i^2*R^3*torque2*sin(PHI_y)*sin(PHI_z) - 16*I_yw^2*L_z_i^2*R^3*torque3*sin(PHI_y)*sin(PHI_z) - 16*I_yw^2*L_z_i^2*R^3*torque4*sin(PHI_y)*sin(PHI_z) + 16*I_yb*I_yw^2*R^2*cos(PHI_y)*X_dot*PHI_z_dot - 16*I_yb*I_yw^2*R^2*sin(PHI_y)*Z_dot*PHI_z_dot - 16*I_yw^2*L_z_i^2*R^3*torque1*cos(PHI_y)*cos(PHI_z)^3 + 16*I_yw^2*L_z_i^2*R^3*torque2*cos(PHI_y)*cos(PHI_z)^3 + 16*I_yw^2*L_z_i^2*R^3*torque3*cos(PHI_y)*cos(PHI_z)^3 - 16*I_yw^2*L_z_i^2*R^3*torque4*cos(PHI_y)*cos(PHI_z)^3 + 16*I_yw^2*R^4*m_b*cos(PHI_y)*X_dot*PHI_z_dot + 64*I_yw^2*R^4*m_w*cos(PHI_y)*X_dot*PHI_z_dot + 16*I_yw^2*L_z_i^2*R^3*torque1*cos(PHI_z)^3*sin(PHI_y) - 16*I_yw^2*L_z_i^2*R^3*torque2*cos(PHI_z)^3*sin(PHI_y) - 16*I_yw^2*L_z_i^2*R^3*torque3*cos(PHI_z)^3*sin(PHI_y) + 16*I_yw^2*L_z_i^2*R^3*torque4*cos(PHI_z)^3*sin(PHI_y) - 16*I_yw^2*R^4*m_b*sin(PHI_y)*Z_dot*PHI_z_dot - 64*I_yw^2*R^4*m_w*sin(PHI_y)*Z_dot*PHI_z_dot + 16*I_yw^2*L_z_i^2*R^3*torque1*sin(PHI_y)*sin(PHI_z)^3 + 16*I_yw^2*L_z_i^2*R^3*torque2*sin(PHI_y)*sin(PHI_z)^3 + 16*I_yw^2*L_z_i^2*R^3*torque3*sin(PHI_y)*sin(PHI_z)^3 + 16*I_yw^2*L_z_i^2*R^3*torque4*sin(PHI_y)*sin(PHI_z)^3 + 64*I_yw^3*L_z_i^2*R^2*cos(PHI_y)*X_dot*PHI_z_dot + 16*I_yw^2*L_z_i^2*R^3*torque1*cos(PHI_y)*cos(PHI_z)^2*sin(PHI_z) + 16*I_yw^2*L_z_i^2*R^3*torque2*cos(PHI_y)*cos(PHI_z)^2*sin(PHI_z) + 16*I_yw^2*L_z_i^2*R^3*torque3*cos(PHI_y)*cos(PHI_z)^2*sin(PHI_z) + 16*I_yw^2*L_z_i^2*R^3*torque4*cos(PHI_y)*cos(PHI_z)^2*sin(PHI_z) - 16*I_yw^2*L_z_i^2*R^2*m_b*cos(PHI_y)*X_dot*PHI_z_dot + 16*I_yw^2*L_z_i^2*R^4*m_b*cos(PHI_y)*X_dot*PHI_z_dot + 64*I_yw^2*L_x_i^2*R^2*m_w*cos(PHI_y)*X_dot*PHI_z_dot + 64*I_yw*L_x_i^2*R^4*m_w^2*cos(PHI_y)*X_dot*PHI_z_dot + 64*I_yw^2*L_y_i^2*R^2*m_w*cos(PHI_y)*X_dot*PHI_z_dot + 64*I_yw*L_y_i^2*R^4*m_w^2*cos(PHI_y)*X_dot*PHI_z_dot + 64*I_yw*L_z_i^2*R^4*m_w^2*cos(PHI_y)*X_dot*PHI_z_dot + 64*I_yw^2*L_z_i^2*R^4*m_w*cos(PHI_y)*X_dot*PHI_z_dot + 16*I_yw^2*L_z_i^2*R^2*m_b*sin(PHI_y)*Z_dot*PHI_z_dot - 16*I_yw^2*L_z_i^2*R^4*m_b*sin(PHI_y)*Z_dot*PHI_z_dot - 64*I_yw^2*L_x_i^2*R^2*m_w*sin(PHI_y)*Z_dot*PHI_z_dot - 64*I_yw*L_x_i^2*R^4*m_w^2*sin(PHI_y)*Z_dot*PHI_z_dot - 64*I_yw^2*L_y_i^2*R^2*m_w*sin(PHI_y)*Z_dot*PHI_z_dot - 64*I_yw*L_y_i^2*R^4*m_w^2*sin(PHI_y)*Z_dot*PHI_z_dot - 64*I_yw*L_z_i^2*R^4*m_w^2*sin(PHI_y)*Z_dot*PHI_z_dot - 64*I_yw^2*L_z_i^2*R^4*m_w*sin(PHI_y)*Z_dot*PHI_z_dot - 64*I_yw^3*L_z_i^2*R^2*cos(PHI_y)*cos(PHI_z)^2*X_dot*PHI_z_dot + 4*I_yb*I_yw*R^4*m_b*cos(PHI_y)*X_dot*PHI_z_dot + 16*I_yb*I_yw*R^4*m_w*cos(PHI_y)*X_dot*PHI_z_dot + 64*I_yw^3*L_z_i^2*R^2*cos(PHI_z)^2*sin(PHI_y)*Z_dot*PHI_z_dot - 4*I_yb*I_yw*R^4*m_b*sin(PHI_y)*Z_dot*PHI_z_dot - 16*I_yb*I_yw*R^4*m_w*sin(PHI_y)*Z_dot*PHI_z_dot - 8*I_yw^2*L_z_i^2*R^4*m_b*sin(2*PHI_z)*diff(Y_w_posi(t), t)*PHI_z_dot - 32*I_yw^2*L_z_i^2*R^4*m_w*sin(2*PHI_z)*diff(Y_w_posi(t), t)*PHI_z_dot + 64*I_yw^3*L_z_i^2*R^2*cos(PHI_y)^2*cos(PHI_z)^2*X_dot*PHI_z_dot - 64*I_yw^3*L_z_i^2*R^2*cos(PHI_y)^2*cos(PHI_z)^2*Z_dot*PHI_z_dot - 16*I_yw^2*L_z_i^2*R^4*m_b*cos(PHI_y)*cos(PHI_z)^2*X_dot*PHI_z_dot - 64*I_yw^2*L_z_i^2*R^4*m_w*cos(PHI_y)*cos(PHI_z)^2*X_dot*PHI_z_dot + 16*I_yw^2*L_z_i^2*R^4*m_b*cos(PHI_z)^2*sin(PHI_y)*Z_dot*PHI_z_dot + 64*I_yw^2*L_z_i^2*R^4*m_w*cos(PHI_z)^2*sin(PHI_y)*Z_dot*PHI_z_dot + 16*I_yw*L_x_i^2*R^4*m_b*m_w*cos(PHI_y)*X_dot*PHI_z_dot + 16*I_yw*L_y_i^2*R^4*m_b*m_w*cos(PHI_y)*X_dot*PHI_z_dot + 16*I_yw*L_z_i^2*R^4*m_b*m_w*cos(PHI_y)*X_dot*PHI_z_dot - 16*I_yw*L_x_i^2*R^4*m_b*m_w*sin(PHI_y)*Z_dot*PHI_z_dot - 16*I_yw*L_y_i^2*R^4*m_b*m_w*sin(PHI_y)*Z_dot*PHI_z_dot - 16*I_yw*L_z_i^2*R^4*m_b*m_w*sin(PHI_y)*Z_dot*PHI_z_dot - 64*I_yw^3*L_z_i^2*R^2*cos(PHI_y)*cos(PHI_z)^2*sin(PHI_y)*X_dot*PHI_z_dot - 64*I_yw^3*L_z_i^2*R^2*cos(PHI_y)*cos(PHI_z)^2*sin(PHI_y)*Z_dot*PHI_z_dot + 16*G*I_yw^2*L_z_i^2*R^4*m_b*cos(PHI_z)*sin(PHI_y)*sin(PHI_z) + 64*G*I_yw^2*L_z_i^2*R^4*m_w*cos(PHI_z)*sin(PHI_y)*sin(PHI_z) + 16*I_yw^2*L_z_i^2*R^4*m_b*cos(PHI_y)*cos(PHI_z)*sin(PHI_z)*Z_dot*PHI_y_dot + 64*I_yw^2*L_z_i^2*R^4*m_w*cos(PHI_y)*cos(PHI_z)*sin(PHI_z)*Z_dot*PHI_y_dot + 16*I_yw^2*L_z_i^2*R^4*m_b*cos(PHI_z)*sin(PHI_y)*sin(PHI_z)*X_dot*PHI_y_dot + 64*I_yw^2*L_z_i^2*R^4*m_w*cos(PHI_z)*sin(PHI_y)*sin(PHI_z)*X_dot*PHI_y_dot)/((4*I_yw + R^2*m_b + 4*R^2*m_w)*(16*I_yw^2*R^2 - 16*I_yw^2*L_z_i^2 + 16*I_yw^2*L_z_i^2*R^2 + 16*L_x_i^2*R^4*m_w^2 + 16*L_y_i^2*R^4*m_w^2 + 16*L_z_i^2*R^4*m_w^2 + 4*I_yb*I_yw*R^2 + I_yb*R^4*m_b + 4*I_yw*R^4*m_b + 4*I_yb*R^4*m_w + 16*I_yw*R^4*m_w - 16*I_yw^2*L_z_i^2*R^2*cos(PHI_z)^2 - 4*I_yw*L_z_i^2*R^2*m_b + 16*I_yw*L_x_i^2*R^2*m_w + 16*I_yw*L_y_i^2*R^2*m_w + 4*L_x_i^2*R^4*m_b*m_w + 4*L_y_i^2*R^4*m_b*m_w + 4*L_z_i^2*R^4*m_b*m_w + 16*I_yw^2*L_z_i^2*R^2*cos(PHI_y)*cos(PHI_z)^2 - 16*I_yw^2*L_z_i^2*R^2*cos(PHI_z)^2*sin(PHI_y)))
Z_dotdot = (64*I_yw^3*L_z_i^2*X_dot*PHI_y_dot - 64*I_yw^3*R^2*X_dot*PHI_y_dot + G*I_yb*R^6*m_b^2 + 16*G*I_yw^2*R^4*m_b + 4*G*I_yw*R^6*m_b^2 + 16*G*I_yb*R^6*m_w^2 + 64*G*I_yw^2*R^4*m_w + 64*G*I_yw*R^6*m_w^2 - 64*G*I_yw^3*L_z_i^2*cos(PHI_y)^2 + 64*G*I_yw^3*R^2*cos(PHI_y)^2 + 64*G*L_x_i^2*R^6*m_w^3 + 64*G*L_y_i^2*R^6*m_w^3 + 64*G*L_z_i^2*R^6*m_w^3 + 16*G*I_yw^2*R^4*m_b*cos(PHI_y)^2 + 64*G*I_yw^2*R^4*m_w*cos(PHI_y)^2 - 16*G*I_yw^2*L_z_i^2*R^2*m_b - 4*G*I_yw*L_z_i^2*R^4*m_b^2 + 16*G*I_yw^2*L_z_i^2*R^4*m_b + 64*G*I_yw*L_x_i^2*R^4*m_w^2 + 64*G*I_yw*L_y_i^2*R^4*m_w^2 - 64*G*I_yw^2*L_z_i^2*R^2*m_w + 64*G*I_yw^2*L_z_i^2*R^4*m_w + 16*I_yw^2*L_z_i^2*R^3*torque1*sin(PHI_z) - 16*I_yw^2*L_z_i^2*R^3*torque2*sin(PHI_z) - 16*I_yw^2*L_z_i^2*R^3*torque3*sin(PHI_z) + 16*I_yw^2*L_z_i^2*R^3*torque4*sin(PHI_z) + 32*G*L_x_i^2*R^6*m_b*m_w^2 + 4*G*L_x_i^2*R^6*m_b^2*m_w + 32*G*L_y_i^2*R^6*m_b*m_w^2 + 4*G*L_y_i^2*R^6*m_b^2*m_w + 32*G*L_z_i^2*R^6*m_b*m_w^2 + 4*G*L_z_i^2*R^6*m_b^2*m_w + 64*G*I_yw^3*L_z_i^2*R^2*cos(PHI_y)^2 - 16*I_yb*I_yw^2*R^2*X_dot*PHI_y_dot - 64*I_yw^3*L_z_i^2*sin(PHI_y)*Y_dot*PHI_z_dot + 4*G*I_yb*I_yw*R^4*m_b + 16*G*I_yb*I_yw*R^4*m_w + 64*I_yw^3*R^2*sin(PHI_y)*Y_dot*PHI_z_dot + 16*I_yw^2*L_z_i^2*R^3*torque1*cos(PHI_z)^3 + 16*I_yw^2*L_z_i^2*R^3*torque2*cos(PHI_z)^3 + 16*I_yw^2*L_z_i^2*R^3*torque3*cos(PHI_z)^3 + 16*I_yw^2*L_z_i^2*R^3*torque4*cos(PHI_z)^3 - 16*I_yw^2*R^4*m_b*X_dot*PHI_y_dot - 64*I_yw^2*R^4*m_w*X_dot*PHI_y_dot + 8*G*I_yb*R^6*m_b*m_w + 32*G*I_yw*R^6*m_b*m_w - 16*I_yw^2*L_z_i^2*R^3*torque1*sin(PHI_z)^3 + 16*I_yw^2*L_z_i^2*R^3*torque2*sin(PHI_z)^3 + 16*I_yw^2*L_z_i^2*R^3*torque3*sin(PHI_z)^3 - 16*I_yw^2*L_z_i^2*R^3*torque4*sin(PHI_z)^3 - 64*I_yw^3*L_z_i^2*cos(PHI_y)^2*X_dot*PHI_y_dot + 64*I_yw^3*R^2*cos(PHI_y)^2*X_dot*PHI_y_dot + 32*I_yw^3*L_z_i^2*sin(2*PHI_y)*Z_dot*PHI_y_dot - 16*I_yw^2*R^3*torque1*cos(PHI_z)*sin(PHI_y) - 16*I_yw^2*R^3*torque2*cos(PHI_z)*sin(PHI_y) - 16*I_yw^2*R^3*torque3*cos(PHI_z)*sin(PHI_y) - 16*I_yw^2*R^3*torque4*cos(PHI_z)*sin(PHI_y) - 32*I_yw^3*R^2*sin(2*PHI_y)*Z_dot*PHI_y_dot - 64*I_yw^3*L_z_i^2*R^2*X_dot*PHI_y_dot - 16*I_yw^2*R^3*torque1*sin(PHI_y)*sin(PHI_z) + 16*I_yw^2*R^3*torque2*sin(PHI_y)*sin(PHI_z) + 16*I_yw^2*R^3*torque3*sin(PHI_y)*sin(PHI_z) - 16*I_yw^2*R^3*torque4*sin(PHI_y)*sin(PHI_z) + 16*G*I_yb*I_yw^2*R^2*cos(PHI_y)^2 - 8*I_yb*I_yw^2*R^2*sin(2*PHI_y)*Z_dot*PHI_y_dot + 16*I_yw^2*L_z_i^2*R*torque1*cos(PHI_z)*sin(PHI_y) + 16*I_yw^2*L_z_i^2*R*torque2*cos(PHI_z)*sin(PHI_y) + 16*I_yw^2*L_z_i^2*R*torque3*cos(PHI_z)*sin(PHI_y) + 16*I_yw^2*L_z_i^2*R*torque4*cos(PHI_z)*sin(PHI_y) + 64*I_yw^3*L_z_i^2*R^2*sin(PHI_y)*Y_dot*PHI_z_dot - 16*I_yw^2*L_z_i^2*R^3*torque1*cos(PHI_y)^2*cos(PHI_z)^3 - 16*I_yw^2*L_z_i^2*R^3*torque2*cos(PHI_y)^2*cos(PHI_z)^3 - 16*I_yw^2*L_z_i^2*R^3*torque3*cos(PHI_y)^2*cos(PHI_z)^3 - 16*I_yw^2*L_z_i^2*R^3*torque4*cos(PHI_y)^2*cos(PHI_z)^3 + 16*I_yw^2*L_z_i^2*R*torque1*sin(PHI_y)*sin(PHI_z) - 16*I_yw^2*L_z_i^2*R*torque2*sin(PHI_y)*sin(PHI_z) - 16*I_yw^2*L_z_i^2*R*torque3*sin(PHI_y)*sin(PHI_z) + 16*I_yw^2*L_z_i^2*R*torque4*sin(PHI_y)*sin(PHI_z) + 16*I_yw^2*R^4*m_b*cos(PHI_y)^2*X_dot*PHI_y_dot + 64*I_yw^2*R^4*m_w*cos(PHI_y)^2*X_dot*PHI_y_dot - 8*I_yw^2*R^4*m_b*sin(2*PHI_y)*Z_dot*PHI_y_dot - 32*I_yw^2*R^4*m_w*sin(2*PHI_y)*Z_dot*PHI_y_dot + 16*I_yw^2*L_z_i^2*R^2*m_b*X_dot*PHI_y_dot - 64*I_yw^2*L_x_i^2*R^2*m_w*X_dot*PHI_y_dot - 64*I_yw*L_x_i^2*R^4*m_w^2*X_dot*PHI_y_dot - 64*I_yw^2*L_y_i^2*R^2*m_w*X_dot*PHI_y_dot - 64*I_yw*L_y_i^2*R^4*m_w^2*X_dot*PHI_y_dot - 64*I_yw*L_z_i^2*R^4*m_w^2*X_dot*PHI_y_dot + 4*I_yw*L_z_i^2*R^5*m_b*torque1*cos(PHI_z) + 4*I_yw*L_z_i^2*R^5*m_b*torque2*cos(PHI_z) + 4*I_yw*L_z_i^2*R^5*m_b*torque3*cos(PHI_z) + 4*I_yw*L_z_i^2*R^5*m_b*torque4*cos(PHI_z) + 16*I_yw*L_z_i^2*R^5*m_w*torque1*cos(PHI_z) + 16*I_yw*L_z_i^2*R^5*m_w*torque2*cos(PHI_z) + 16*I_yw*L_z_i^2*R^5*m_w*torque3*cos(PHI_z) + 16*I_yw*L_z_i^2*R^5*m_w*torque4*cos(PHI_z) + 16*G*I_yw*L_x_i^2*R^4*m_b*m_w + 16*G*I_yw*L_y_i^2*R^4*m_b*m_w - 16*G*I_yw*L_z_i^2*R^4*m_b*m_w + 64*I_yw^3*L_z_i^2*R^2*cos(PHI_y)^2*X_dot*PHI_y_dot + 64*I_yw^3*L_z_i^2*R^2*cos(PHI_z)^2*X_dot*PHI_y_dot - 64*I_yw^3*L_z_i^2*R^2*cos(PHI_z)^2*Y_dot*PHI_z_dot - 16*I_yw^2*L_z_i^2*R^3*torque1*cos(PHI_z)*sin(PHI_y) - 16*I_yw^2*L_z_i^2*R^3*torque2*cos(PHI_z)*sin(PHI_y) - 16*I_yw^2*L_z_i^2*R^3*torque3*cos(PHI_z)*sin(PHI_y) - 16*I_yw^2*L_z_i^2*R^3*torque4*cos(PHI_z)*sin(PHI_y) - 32*I_yw^3*L_z_i^2*R^2*sin(2*PHI_y)*Z_dot*PHI_y_dot - 4*I_yb*I_yw*R^4*m_b*X_dot*PHI_y_dot - 16*I_yb*I_yw*R^4*m_w*X_dot*PHI_y_dot + 64*G*I_yw^3*L_z_i^2*R^2*cos(PHI_y)*cos(PHI_z)^2 - 16*L_x_i^2*R^5*m_w^2*torque1*cos(PHI_z)*sin(PHI_y) - 16*L_x_i^2*R^5*m_w^2*torque2*cos(PHI_z)*sin(PHI_y) - 16*L_x_i^2*R^5*m_w^2*torque3*cos(PHI_z)*sin(PHI_y) - 16*L_x_i^2*R^5*m_w^2*torque4*cos(PHI_z)*sin(PHI_y) - 16*L_y_i^2*R^5*m_w^2*torque1*cos(PHI_z)*sin(PHI_y) - 16*L_y_i^2*R^5*m_w^2*torque2*cos(PHI_z)*sin(PHI_y) - 16*L_y_i^2*R^5*m_w^2*torque3*cos(PHI_z)*sin(PHI_y) - 16*L_y_i^2*R^5*m_w^2*torque4*cos(PHI_z)*sin(PHI_y) - 16*L_z_i^2*R^5*m_w^2*torque1*cos(PHI_z)*sin(PHI_y) - 16*L_z_i^2*R^5*m_w^2*torque2*cos(PHI_z)*sin(PHI_y) - 16*L_z_i^2*R^5*m_w^2*torque3*cos(PHI_z)*sin(PHI_y) - 16*L_z_i^2*R^5*m_w^2*torque4*cos(PHI_z)*sin(PHI_y) - 16*L_x_i^2*R^5*m_w^2*torque1*sin(PHI_y)*sin(PHI_z) + 16*L_x_i^2*R^5*m_w^2*torque2*sin(PHI_y)*sin(PHI_z) + 16*L_x_i^2*R^5*m_w^2*torque3*sin(PHI_y)*sin(PHI_z) - 16*L_x_i^2*R^5*m_w^2*torque4*sin(PHI_y)*sin(PHI_z) - 16*L_y_i^2*R^5*m_w^2*torque1*sin(PHI_y)*sin(PHI_z) + 16*L_y_i^2*R^5*m_w^2*torque2*sin(PHI_y)*sin(PHI_z) + 16*L_y_i^2*R^5*m_w^2*torque3*sin(PHI_y)*sin(PHI_z) - 16*L_y_i^2*R^5*m_w^2*torque4*sin(PHI_y)*sin(PHI_z) - 16*L_z_i^2*R^5*m_w^2*torque1*sin(PHI_y)*sin(PHI_z) + 16*L_z_i^2*R^5*m_w^2*torque2*sin(PHI_y)*sin(PHI_z) + 16*L_z_i^2*R^5*m_w^2*torque3*sin(PHI_y)*sin(PHI_z) - 16*L_z_i^2*R^5*m_w^2*torque4*sin(PHI_y)*sin(PHI_z) - 4*I_yb*I_yw*R^3*torque1*cos(PHI_z)*sin(PHI_y) - 4*I_yb*I_yw*R^3*torque2*cos(PHI_z)*sin(PHI_y) - 4*I_yb*I_yw*R^3*torque3*cos(PHI_z)*sin(PHI_y) - 4*I_yb*I_yw*R^3*torque4*cos(PHI_z)*sin(PHI_y) + 16*I_yb*I_yw^2*R^2*sin(PHI_y)*Y_dot*PHI_z_dot - 4*I_yb*I_yw*R^3*torque1*sin(PHI_y)*sin(PHI_z) + 4*I_yb*I_yw*R^3*torque2*sin(PHI_y)*sin(PHI_z) + 4*I_yb*I_yw*R^3*torque3*sin(PHI_y)*sin(PHI_z) - 4*I_yb*I_yw*R^3*torque4*sin(PHI_y)*sin(PHI_z) + 16*I_yw^2*L_z_i^2*R^3*torque1*cos(PHI_y)^2*cos(PHI_z) + 16*I_yw^2*L_z_i^2*R^3*torque2*cos(PHI_y)^2*cos(PHI_z) + 16*I_yw^2*L_z_i^2*R^3*torque3*cos(PHI_y)^2*cos(PHI_z) + 16*I_yw^2*L_z_i^2*R^3*torque4*cos(PHI_y)^2*cos(PHI_z) - 16*G*I_yw^2*L_z_i^2*R^2*m_b*cos(PHI_y)^2 + 64*G*I_yw^2*L_x_i^2*R^2*m_w*cos(PHI_y)^2 + 64*G*I_yw*L_x_i^2*R^4*m_w^2*cos(PHI_y)^2 + 64*G*I_yw^2*L_y_i^2*R^2*m_w*cos(PHI_y)^2 + 64*G*I_yw*L_y_i^2*R^4*m_w^2*cos(PHI_y)^2 + 64*G*I_yw*L_z_i^2*R^4*m_w^2*cos(PHI_y)^2 - 16*G*I_yw^2*L_z_i^2*R^4*m_b*cos(PHI_z)^2 - 64*G*I_yw^2*L_z_i^2*R^4*m_w*cos(PHI_z)^2 + 16*I_yw^2*L_z_i^2*R^3*torque1*cos(PHI_z)^3*sin(PHI_y) + 16*I_yw^2*L_z_i^2*R^3*torque2*cos(PHI_z)^3*sin(PHI_y) + 16*I_yw^2*L_z_i^2*R^3*torque3*cos(PHI_z)^3*sin(PHI_y) + 16*I_yw^2*L_z_i^2*R^3*torque4*cos(PHI_z)^3*sin(PHI_y) - I_yb*R^5*m_b*torque1*cos(PHI_z)*sin(PHI_y) - I_yb*R^5*m_b*torque2*cos(PHI_z)*sin(PHI_y) - I_yb*R^5*m_b*torque3*cos(PHI_z)*sin(PHI_y) - I_yb*R^5*m_b*torque4*cos(PHI_z)*sin(PHI_y) - 4*I_yw*R^5*m_b*torque1*cos(PHI_z)*sin(PHI_y) - 4*I_yw*R^5*m_b*torque2*cos(PHI_z)*sin(PHI_y) - 4*I_yw*R^5*m_b*torque3*cos(PHI_z)*sin(PHI_y) - 4*I_yw*R^5*m_b*torque4*cos(PHI_z)*sin(PHI_y) - 4*I_yb*R^5*m_w*torque1*cos(PHI_z)*sin(PHI_y) - 4*I_yb*R^5*m_w*torque2*cos(PHI_z)*sin(PHI_y) - 4*I_yb*R^5*m_w*torque3*cos(PHI_z)*sin(PHI_y) - 4*I_yb*R^5*m_w*torque4*cos(PHI_z)*sin(PHI_y) - 16*I_yw*R^5*m_w*torque1*cos(PHI_z)*sin(PHI_y) - 16*I_yw*R^5*m_w*torque2*cos(PHI_z)*sin(PHI_y) - 16*I_yw*R^5*m_w*torque3*cos(PHI_z)*sin(PHI_y) - 16*I_yw*R^5*m_w*torque4*cos(PHI_z)*sin(PHI_y) + 16*I_yw^2*R^4*m_b*sin(PHI_y)*Y_dot*PHI_z_dot + 64*I_yw^2*R^4*m_w*sin(PHI_y)*Y_dot*PHI_z_dot - 16*I_yw^2*L_z_i^2*R^3*torque1*sin(PHI_y)*sin(PHI_z)^3 + 16*I_yw^2*L_z_i^2*R^3*torque2*sin(PHI_y)*sin(PHI_z)^3 + 16*I_yw^2*L_z_i^2*R^3*torque3*sin(PHI_y)*sin(PHI_z)^3 - 16*I_yw^2*L_z_i^2*R^3*torque4*sin(PHI_y)*sin(PHI_z)^3 - I_yb*R^5*m_b*torque1*sin(PHI_y)*sin(PHI_z) + I_yb*R^5*m_b*torque2*sin(PHI_y)*sin(PHI_z) + I_yb*R^5*m_b*torque3*sin(PHI_y)*sin(PHI_z) - I_yb*R^5*m_b*torque4*sin(PHI_y)*sin(PHI_z) - 4*I_yw*R^5*m_b*torque1*sin(PHI_y)*sin(PHI_z) + 4*I_yw*R^5*m_b*torque2*sin(PHI_y)*sin(PHI_z) + 4*I_yw*R^5*m_b*torque3*sin(PHI_y)*sin(PHI_z) - 4*I_yw*R^5*m_b*torque4*sin(PHI_y)*sin(PHI_z) - 4*I_yb*R^5*m_w*torque1*sin(PHI_y)*sin(PHI_z) + 4*I_yb*R^5*m_w*torque2*sin(PHI_y)*sin(PHI_z) + 4*I_yb*R^5*m_w*torque3*sin(PHI_y)*sin(PHI_z) - 4*I_yb*R^5*m_w*torque4*sin(PHI_y)*sin(PHI_z) - 16*I_yw*R^5*m_w*torque1*sin(PHI_y)*sin(PHI_z) + 16*I_yw*R^5*m_w*torque2*sin(PHI_y)*sin(PHI_z) + 16*I_yw*R^5*m_w*torque3*sin(PHI_y)*sin(PHI_z) - 16*I_yw*R^5*m_w*torque4*sin(PHI_y)*sin(PHI_z) - 64*G*I_yw^3*L_z_i^2*R^2*cos(PHI_y)^2*cos(PHI_z)^2 + 16*I_yb*I_yw^2*R^2*cos(PHI_y)^2*X_dot*PHI_y_dot + 4*G*I_yb*I_yw*R^4*m_b*cos(PHI_y)^2 + 16*G*I_yb*I_yw*R^4*m_w*cos(PHI_y)^2 - 2*I_yb*I_yw*R^4*m_b*sin(2*PHI_y)*Z_dot*PHI_y_dot - 8*I_yb*I_yw*R^4*m_w*sin(2*PHI_y)*Z_dot*PHI_y_dot - 16*I_yw*L_x_i^2*R^4*m_b*m_w*X_dot*PHI_y_dot - 16*I_yw*L_y_i^2*R^4*m_b*m_w*X_dot*PHI_y_dot - 16*I_yw*L_z_i^2*R^4*m_b*m_w*X_dot*PHI_y_dot - 16*I_yw^2*L_z_i^2*R^3*torque1*cos(PHI_y)^2*cos(PHI_z)^2*sin(PHI_z) + 16*I_yw^2*L_z_i^2*R^3*torque2*cos(PHI_y)^2*cos(PHI_z)^2*sin(PHI_z) + 16*I_yw^2*L_z_i^2*R^3*torque3*cos(PHI_y)^2*cos(PHI_z)^2*sin(PHI_z) - 16*I_yw^2*L_z_i^2*R^3*torque4*cos(PHI_y)^2*cos(PHI_z)^2*sin(PHI_z) + 4*I_yw*L_z_i^2*R^3*m_b*torque1*cos(PHI_z)*sin(PHI_y) + 4*I_yw*L_z_i^2*R^3*m_b*torque2*cos(PHI_z)*sin(PHI_y) + 4*I_yw*L_z_i^2*R^3*m_b*torque3*cos(PHI_z)*sin(PHI_y) + 4*I_yw*L_z_i^2*R^3*m_b*torque4*cos(PHI_z)*sin(PHI_y) - 16*I_yw*L_x_i^2*R^3*m_w*torque1*cos(PHI_z)*sin(PHI_y) - 16*I_yw*L_x_i^2*R^3*m_w*torque2*cos(PHI_z)*sin(PHI_y) - 16*I_yw*L_x_i^2*R^3*m_w*torque3*cos(PHI_z)*sin(PHI_y) - 16*I_yw*L_x_i^2*R^3*m_w*torque4*cos(PHI_z)*sin(PHI_y) - 16*I_yw*L_y_i^2*R^3*m_w*torque1*cos(PHI_z)*sin(PHI_y) - 16*I_yw*L_y_i^2*R^3*m_w*torque2*cos(PHI_z)*sin(PHI_y) - 16*I_yw*L_y_i^2*R^3*m_w*torque3*cos(PHI_z)*sin(PHI_y) - 16*I_yw*L_y_i^2*R^3*m_w*torque4*cos(PHI_z)*sin(PHI_y) - 16*I_yw^2*L_z_i^2*R^2*m_b*sin(PHI_y)*Y_dot*PHI_z_dot + 64*I_yw^2*L_x_i^2*R^2*m_w*sin(PHI_y)*Y_dot*PHI_z_dot + 64*I_yw*L_x_i^2*R^4*m_w^2*sin(PHI_y)*Y_dot*PHI_z_dot + 64*I_yw^2*L_y_i^2*R^2*m_w*sin(PHI_y)*Y_dot*PHI_z_dot + 64*I_yw*L_y_i^2*R^4*m_w^2*sin(PHI_y)*Y_dot*PHI_z_dot + 64*I_yw*L_z_i^2*R^4*m_w^2*sin(PHI_y)*Y_dot*PHI_z_dot + 4*I_yw*L_z_i^2*R^3*m_b*torque1*sin(PHI_y)*sin(PHI_z) - 4*I_yw*L_z_i^2*R^3*m_b*torque2*sin(PHI_y)*sin(PHI_z) - 4*I_yw*L_z_i^2*R^3*m_b*torque3*sin(PHI_y)*sin(PHI_z) + 4*I_yw*L_z_i^2*R^3*m_b*torque4*sin(PHI_y)*sin(PHI_z) - 16*I_yw*L_x_i^2*R^3*m_w*torque1*sin(PHI_y)*sin(PHI_z) + 16*I_yw*L_x_i^2*R^3*m_w*torque2*sin(PHI_y)*sin(PHI_z) + 16*I_yw*L_x_i^2*R^3*m_w*torque3*sin(PHI_y)*sin(PHI_z) - 16*I_yw*L_x_i^2*R^3*m_w*torque4*sin(PHI_y)*sin(PHI_z) - 16*I_yw*L_y_i^2*R^3*m_w*torque1*sin(PHI_y)*sin(PHI_z) + 16*I_yw*L_y_i^2*R^3*m_w*torque2*sin(PHI_y)*sin(PHI_z) + 16*I_yw*L_y_i^2*R^3*m_w*torque3*sin(PHI_y)*sin(PHI_z) - 16*I_yw*L_y_i^2*R^3*m_w*torque4*sin(PHI_y)*sin(PHI_z) + 64*I_yw^3*L_z_i^2*R^2*cos(PHI_y)*cos(PHI_z)^2*Z_dot*PHI_y_dot - 4*L_x_i^2*R^5*m_b*m_w*torque1*cos(PHI_z)*sin(PHI_y) - 4*L_x_i^2*R^5*m_b*m_w*torque2*cos(PHI_z)*sin(PHI_y) - 4*L_x_i^2*R^5*m_b*m_w*torque3*cos(PHI_z)*sin(PHI_y) - 4*L_x_i^2*R^5*m_b*m_w*torque4*cos(PHI_z)*sin(PHI_y) - 4*L_y_i^2*R^5*m_b*m_w*torque1*cos(PHI_z)*sin(PHI_y) - 4*L_y_i^2*R^5*m_b*m_w*torque2*cos(PHI_z)*sin(PHI_y) - 4*L_y_i^2*R^5*m_b*m_w*torque3*cos(PHI_z)*sin(PHI_y) - 4*L_y_i^2*R^5*m_b*m_w*torque4*cos(PHI_z)*sin(PHI_y) - 4*L_z_i^2*R^5*m_b*m_w*torque1*cos(PHI_z)*sin(PHI_y) - 4*L_z_i^2*R^5*m_b*m_w*torque2*cos(PHI_z)*sin(PHI_y) - 4*L_z_i^2*R^5*m_b*m_w*torque3*cos(PHI_z)*sin(PHI_y) - 4*L_z_i^2*R^5*m_b*m_w*torque4*cos(PHI_z)*sin(PHI_y) + 16*I_yw^2*L_z_i^2*R^3*torque1*cos(PHI_y)*cos(PHI_z)*sin(PHI_y) + 16*I_yw^2*L_z_i^2*R^3*torque2*cos(PHI_y)*cos(PHI_z)*sin(PHI_y) + 16*I_yw^2*L_z_i^2*R^3*torque3*cos(PHI_y)*cos(PHI_z)*sin(PHI_y) + 16*I_yw^2*L_z_i^2*R^3*torque4*cos(PHI_y)*cos(PHI_z)*sin(PHI_y) + 64*I_yw^3*L_z_i^2*R^2*cos(PHI_z)^2*sin(PHI_y)*X_dot*PHI_y_dot - 4*L_x_i^2*R^5*m_b*m_w*torque1*sin(PHI_y)*sin(PHI_z) + 4*L_x_i^2*R^5*m_b*m_w*torque2*sin(PHI_y)*sin(PHI_z) + 4*L_x_i^2*R^5*m_b*m_w*torque3*sin(PHI_y)*sin(PHI_z) - 4*L_x_i^2*R^5*m_b*m_w*torque4*sin(PHI_y)*sin(PHI_z) - 4*L_y_i^2*R^5*m_b*m_w*torque1*sin(PHI_y)*sin(PHI_z) + 4*L_y_i^2*R^5*m_b*m_w*torque2*sin(PHI_y)*sin(PHI_z) + 4*L_y_i^2*R^5*m_b*m_w*torque3*sin(PHI_y)*sin(PHI_z) - 4*L_y_i^2*R^5*m_b*m_w*torque4*sin(PHI_y)*sin(PHI_z) - 4*L_z_i^2*R^5*m_b*m_w*torque1*sin(PHI_y)*sin(PHI_z) + 4*L_z_i^2*R^5*m_b*m_w*torque2*sin(PHI_y)*sin(PHI_z) + 4*L_z_i^2*R^5*m_b*m_w*torque3*sin(PHI_y)*sin(PHI_z) - 4*L_z_i^2*R^5*m_b*m_w*torque4*sin(PHI_y)*sin(PHI_z) - 64*I_yw^3*L_z_i^2*R^2*cos(PHI_z)^2*sin(PHI_y)*Y_dot*PHI_z_dot + 4*I_yb*I_yw*R^4*m_b*sin(PHI_y)*Y_dot*PHI_z_dot + 16*I_yb*I_yw*R^4*m_w*sin(PHI_y)*Y_dot*PHI_z_dot - 16*I_yw^2*L_z_i^2*R^2*m_b*cos(PHI_y)^2*X_dot*PHI_y_dot + 64*I_yw^2*L_x_i^2*R^2*m_w*cos(PHI_y)^2*X_dot*PHI_y_dot + 64*I_yw*L_x_i^2*R^4*m_w^2*cos(PHI_y)^2*X_dot*PHI_y_dot + 64*I_yw^2*L_y_i^2*R^2*m_w*cos(PHI_y)^2*X_dot*PHI_y_dot + 64*I_yw*L_y_i^2*R^4*m_w^2*cos(PHI_y)^2*X_dot*PHI_y_dot + 64*I_yw*L_z_i^2*R^4*m_w^2*cos(PHI_y)^2*X_dot*PHI_y_dot + 16*G*I_yw*L_x_i^2*R^4*m_b*m_w*cos(PHI_y)^2 + 16*G*I_yw*L_y_i^2*R^4*m_b*m_w*cos(PHI_y)^2 + 16*G*I_yw*L_z_i^2*R^4*m_b*m_w*cos(PHI_y)^2 - 16*I_yw^2*L_z_i^2*R^4*m_b*cos(PHI_z)^2*Y_dot*PHI_z_dot - 64*I_yw^2*L_z_i^2*R^4*m_w*cos(PHI_z)^2*Y_dot*PHI_z_dot + 8*I_yw^2*L_z_i^2*R^2*m_b*sin(2*PHI_y)*Z_dot*PHI_y_dot - 32*I_yw^2*L_x_i^2*R^2*m_w*sin(2*PHI_y)*Z_dot*PHI_y_dot - 32*I_yw*L_x_i^2*R^4*m_w^2*sin(2*PHI_y)*Z_dot*PHI_y_dot - 32*I_yw^2*L_y_i^2*R^2*m_w*sin(2*PHI_y)*Z_dot*PHI_y_dot - 32*I_yw*L_y_i^2*R^4*m_w^2*sin(2*PHI_y)*Z_dot*PHI_y_dot - 32*I_yw*L_z_i^2*R^4*m_w^2*sin(2*PHI_y)*Z_dot*PHI_y_dot - 64*I_yw^3*L_z_i^2*R^2*cos(PHI_y)^2*cos(PHI_z)^2*X_dot*PHI_y_dot + 16*G*I_yw^2*L_z_i^2*R^4*m_b*cos(PHI_y)*cos(PHI_z)^2 + 64*G*I_yw^2*L_z_i^2*R^4*m_w*cos(PHI_y)*cos(PHI_z)^2 - 16*I_yw^2*L_z_i^2*R^3*torque1*cos(PHI_y)*cos(PHI_z)^3*sin(PHI_y) - 16*I_yw^2*L_z_i^2*R^3*torque2*cos(PHI_y)*cos(PHI_z)^3*sin(PHI_y) - 16*I_yw^2*L_z_i^2*R^3*torque3*cos(PHI_y)*cos(PHI_z)^3*sin(PHI_y) - 16*I_yw^2*L_z_i^2*R^3*torque4*cos(PHI_y)*cos(PHI_z)^3*sin(PHI_y) + 4*I_yb*I_yw*R^4*m_b*cos(PHI_y)^2*X_dot*PHI_y_dot + 16*I_yb*I_yw*R^4*m_w*cos(PHI_y)^2*X_dot*PHI_y_dot + 16*I_yw^2*L_z_i^2*R^4*m_b*cos(PHI_y)*cos(PHI_z)^2*Z_dot*PHI_y_dot + 64*I_yw^2*L_z_i^2*R^4*m_w*cos(PHI_y)*cos(PHI_z)^2*Z_dot*PHI_y_dot + 16*I_yw^2*L_z_i^2*R^4*m_b*cos(PHI_z)^2*sin(PHI_y)*X_dot*PHI_y_dot + 64*I_yw^2*L_z_i^2*R^4*m_w*cos(PHI_z)^2*sin(PHI_y)*X_dot*PHI_y_dot - 16*I_yw^2*L_z_i^2*R^3*torque1*cos(PHI_y)*cos(PHI_z)^2*sin(PHI_y)*sin(PHI_z) + 16*I_yw^2*L_z_i^2*R^3*torque2*cos(PHI_y)*cos(PHI_z)^2*sin(PHI_y)*sin(PHI_z) + 16*I_yw^2*L_z_i^2*R^3*torque3*cos(PHI_y)*cos(PHI_z)^2*sin(PHI_y)*sin(PHI_z) - 16*I_yw^2*L_z_i^2*R^3*torque4*cos(PHI_y)*cos(PHI_z)^2*sin(PHI_y)*sin(PHI_z) + 16*I_yw*L_x_i^2*R^4*m_b*m_w*sin(PHI_y)*Y_dot*PHI_z_dot + 16*I_yw*L_y_i^2*R^4*m_b*m_w*sin(PHI_y)*Y_dot*PHI_z_dot + 16*I_yw*L_z_i^2*R^4*m_b*m_w*sin(PHI_y)*Y_dot*PHI_z_dot - 64*I_yw^3*L_z_i^2*R^2*cos(PHI_y)*cos(PHI_z)*sin(PHI_z)*Z_dot*PHI_z_dot + 16*I_yw*L_x_i^2*R^4*m_b*m_w*cos(PHI_y)^2*X_dot*PHI_y_dot + 16*I_yw*L_y_i^2*R^4*m_b*m_w*cos(PHI_y)^2*X_dot*PHI_y_dot + 16*I_yw*L_z_i^2*R^4*m_b*m_w*cos(PHI_y)^2*X_dot*PHI_y_dot + 64*I_yw^3*L_z_i^2*R^2*cos(PHI_y)*cos(PHI_z)^2*sin(PHI_y)*Z_dot*PHI_y_dot - 8*I_yw*L_x_i^2*R^4*m_b*m_w*sin(2*PHI_y)*Z_dot*PHI_y_dot - 8*I_yw*L_y_i^2*R^4*m_b*m_w*sin(2*PHI_y)*Z_dot*PHI_y_dot - 8*I_yw*L_z_i^2*R^4*m_b*m_w*sin(2*PHI_y)*Z_dot*PHI_y_dot + 64*I_yw^3*L_z_i^2*R^2*cos(PHI_y)^3*cos(PHI_z)*sin(PHI_z)*X_dot*PHI_z_dot + 64*I_yw^3*L_z_i^2*R^2*cos(PHI_y)^3*cos(PHI_z)*sin(PHI_z)*Z_dot*PHI_z_dot - 16*I_yw^2*L_z_i^2*R^4*m_b*cos(PHI_z)*sin(PHI_y)*sin(PHI_z)*Z_dot*PHI_z_dot - 64*I_yw^2*L_z_i^2*R^4*m_w*cos(PHI_z)*sin(PHI_y)*sin(PHI_z)*Z_dot*PHI_z_dot + 64*I_yw^3*L_z_i^2*R^2*cos(PHI_y)^2*cos(PHI_z)*sin(PHI_y)*sin(PHI_z)*X_dot*PHI_z_dot - 64*I_yw^3*L_z_i^2*R^2*cos(PHI_y)^2*cos(PHI_z)*sin(PHI_y)*sin(PHI_z)*Z_dot*PHI_z_dot + 16*I_yw^2*L_z_i^2*R^4*m_b*cos(PHI_y)*cos(PHI_z)*sin(PHI_z)*X_dot*PHI_z_dot + 64*I_yw^2*L_z_i^2*R^4*m_w*cos(PHI_y)*cos(PHI_z)*sin(PHI_z)*X_dot*PHI_z_dot)/((4*I_yw + R^2*m_b + 4*R^2*m_w)*(16*I_yw^2*R^2 - 16*I_yw^2*L_z_i^2 + 16*I_yw^2*L_z_i^2*R^2 + 16*L_x_i^2*R^4*m_w^2 + 16*L_y_i^2*R^4*m_w^2 + 16*L_z_i^2*R^4*m_w^2 + 4*I_yb*I_yw*R^2 + I_yb*R^4*m_b + 4*I_yw*R^4*m_b + 4*I_yb*R^4*m_w + 16*I_yw*R^4*m_w - 16*I_yw^2*L_z_i^2*R^2*cos(PHI_z)^2 - 4*I_yw*L_z_i^2*R^2*m_b + 16*I_yw*L_x_i^2*R^2*m_w + 16*I_yw*L_y_i^2*R^2*m_w + 4*L_x_i^2*R^4*m_b*m_w + 4*L_y_i^2*R^4*m_b*m_w + 4*L_z_i^2*R^4*m_b*m_w + 16*I_yw^2*L_z_i^2*R^2*cos(PHI_y)*cos(PHI_z)^2 - 16*I_yw^2*L_z_i^2*R^2*cos(PHI_z)^2*sin(PHI_y)))
 
PHI_y_dotdot = -(L_z_i*R^2*(m_b + 4*m_w)*(R*torque1 + R*torque2 + R*torque3 + R*torque4 - 4*I_yw*cos(PHI_z)*Y_dot*PHI_z_dot + 4*G*I_yw*cos(PHI_z)*sin(PHI_y) + 4*I_yw*cos(PHI_y)*cos(PHI_z)*Z_dot*PHI_y_dot + 4*I_yw*cos(PHI_z)*sin(PHI_y)*X_dot*PHI_y_dot + 4*I_yw*cos(PHI_y)*sin(PHI_z)*X_dot*PHI_z_dot - 4*I_yw*sin(PHI_y)*sin(PHI_z)*Z_dot*PHI_z_dot))/(16*I_yw^2*R^2 - 16*I_yw^2*L_z_i^2 + 16*I_yw^2*L_z_i^2*R^2 + 16*L_x_i^2*R^4*m_w^2 + 16*L_y_i^2*R^4*m_w^2 + 16*L_z_i^2*R^4*m_w^2 + 4*I_yb*I_yw*R^2 + I_yb*R^4*m_b + 4*I_yw*R^4*m_b + 4*I_yb*R^4*m_w + 16*I_yw*R^4*m_w - 16*I_yw^2*L_z_i^2*R^2*cos(PHI_z)^2 - 4*I_yw*L_z_i^2*R^2*m_b + 16*I_yw*L_x_i^2*R^2*m_w + 16*I_yw*L_y_i^2*R^2*m_w + 4*L_x_i^2*R^4*m_b*m_w + 4*L_y_i^2*R^4*m_b*m_w + 4*L_z_i^2*R^4*m_b*m_w + 16*I_yw^2*L_z_i^2*R^2*cos(PHI_y)*cos(PHI_z)^2 - 16*I_yw^2*L_z_i^2*R^2*cos(PHI_z)^2*sin(PHI_y)); 
PHI_z_dotdot = -(R*(L_x_i + L_y_i)*(torque1 - torque2 + torque3 - torque4))/(4*I_yw*L_x_i^2 + 4*I_yw*L_y_i^2 + I_zb*R^2 + 4*I_zw*R^2 + 4*L_x_i^2*R^2*m_w + 4*L_y_i^2*R^2*m_w + 4*L_z_i^2*R^2*m_w + 8*I_yw*L_x_i*L_y_i);

167
X_dot = X_dot + X_dotdot*dt;
Y_dot = Y_dot + Y_dotdot*dt;
Z_dot = Z_dot + Z_dotdot*dt;

PHI_y_dot = PHI_y_dot + PHI_y_dotdot *dt;
PHI_z_dot = PHI_z_dot + PHI_z_dotdot *dt;

X = X + X_dot*dt;
Y = Y + Y_dot*dt;
Z = Z + Z_dot*dt;
PHI_x = PHI_x + PHI_x_dot *dt;
PHI_y = PHI_y + PHI_y_dot *dt;
PHI_z = PHI_z + PHI_z_dot *dt;
